simulink model "truesystem"  (R2020a)
settings: Solver=VariableStepAuto  StartTime=0.0  StopTime=stoptimetotal  RelTol=1e-3
values from neighbouring files (symbols this model uses):
  battery = load('params/battery.mat').battery    [prognostics.m]    (also in workspace_1.mat = )
  IC = load('params/IC_HoverAt10ftOcto.mat').IC    [prognostics.m]    (also in workspace_1.mat = )
  Motor1 = load('params/Motors/Motor1.mat').Motor    [prognostics.m]    (also in workspace_1.mat = )
  Motor2 = load('params/Motors/Motor2.mat').Motor    [prognostics.m]    (also in workspace_1.mat = )
  Motor3 = load('params/Motors/Motor3.mat').Motor    [prognostics.m]    (also in workspace_1.mat = )
  Motor4 = load('params/Motors/Motor4.mat').Motor    [prognostics.m]    (also in workspace_1.mat = )
  Motor5 = load('params/Motors/Motor5.mat').Motor    [prognostics.m]    (also in workspace_1.mat = )
  Motor6 = load('params/Motors/Motor6.mat').Motor    [prognostics.m]    (also in workspace_1.mat = )
  Motor7 = load('params/Motors/Motor7.mat').Motor    [prognostics.m]    (also in workspace_1.mat = )
  Motor8 = load('params/Motors/Motor8.mat').Motor    [prognostics.m]    (also in workspace_1.mat = )
  octomodel = load('params/octoModel.mat').octomodel    [prognostics.m]    (also in workspace_1.mat = )
  sampletimetraj = 1    [prognostics.m]    (also in workspace_1.mat)
undefined symbols (not defined in the file or in its folder): DiscIntNeverNeededParam, mu_wind
libraries: dspstat3 x9, sharedTrackingLibrary x4
(part 2 of 2)

== system truesystem/Motors/DC Motor 3/Mechanical part ==
  Static Friction Torque : Inport
  Electrical Torque : Inport  Port=2
  1/J Inertia constant : Gain  Gain=1/Motor3.J
  "Df viscous damping coefficient Dynamic Friction coefficient " : Gain  Gain=Motor3.Df
  Discrete-Time Integrator : DiscreteIntegrator  gainval=1  InitialCondition=IC.w3  SampleTime=octomodel.sampletime  ICPrevOutput=DiscIntNeverNeededParam  ICPrevScaledInput=DiscIntNeverNeededParam
  Gain : Gain  Gain=Motor3.cq
  Square : Math  Operator=square  SaturateOnIntegerOverflow=on
  Sum1 : Sum  Inputs=--+-
  w angular speed : Outport  VectorParamsAs1DForOutWhenUnconnected=off
  Torque : Outport  Port=2  VectorParamsAs1DForOutWhenUnconnected=off
  wires:
  1/J Inertia constant/1 -> Discrete-Time Integrator/1
  Static Friction Torque/1 -> Sum1/2
  "Df viscous damping coefficient Dynamic Friction coefficient "/1 -> Sum1/4
  Discrete-Time Integrator/1 -> w angular speed/1, Square/1, "Df viscous damping coefficient Dynamic Friction coefficient "/1  "w angular speed"
  Sum1/1 -> 1/J Inertia constant/1
  Electrical Torque/1 -> Sum1/3
  Gain/1 -> Torque/1, Sum1/1
  Square/1 -> Gain/1

== system truesystem/Motors/DC Motor 4/Electrical part ==
  ESC voltage : Inport
  w angular speed : Inport  Port=2
  1/R : Gain  Gain=1/Motor2.Req
  Ke (Torque constant)1 : Gain  Gain=Motor2.Ke_eq
  Kt (Torque constant) Kt=Ke for an ideal square wave motor : Gain  Gain=Motor2.Ke_eq
  Saturation : Saturate  UpperLimit=11  LowerLimit=0
  Scope1 : Scope
  Scope2 : Scope
  Scope3 : Scope
  Sum : Sum  Inputs=|+-
  Electrical Torque : Outport  VectorParamsAs1DForOutWhenUnconnected=off
  current : Outport  Port=2  VectorParamsAs1DForOutWhenUnconnected=off
  wires:
  Saturation/1 -> current/1, Kt (Torque constant) Kt=Ke for an ideal square wave motor/1, Scope1/1
  w angular speed/1 -> Ke (Torque constant)1/1
  ESC voltage/1 -> Sum/1
  Ke (Torque constant)1/1 -> Sum/2, Scope2/1
  Kt (Torque constant) Kt=Ke for an ideal square wave motor/1 -> Electrical Torque/1
  Sum/1 -> 1/R/1, Scope3/1
  1/R/1 -> Saturation/1  "current i"

== system truesystem/Motors/DC Motor 4/Mechanical part ==
  Static Friction Torque : Inport
  Electrical Torque : Inport  Port=2
  1/J Inertia constant : Gain  Gain=1/Motor2.J
  "Df viscous damping coefficient Dynamic Friction coefficient " : Gain  Gain=Motor2.Df
  Discrete-Time Integrator : DiscreteIntegrator  gainval=1  InitialCondition=IC.w2  SampleTime=octomodel.sampletime  ICPrevOutput=DiscIntNeverNeededParam  ICPrevScaledInput=DiscIntNeverNeededParam
  Gain : Gain  Gain=Motor2.cq
  Square : Math  Operator=square  SaturateOnIntegerOverflow=on
  Sum1 : Sum  Inputs=--+-
  w angular speed : Outport  VectorParamsAs1DForOutWhenUnconnected=off
  Torque : Outport  Port=2  VectorParamsAs1DForOutWhenUnconnected=off
  wires:
  Square/1 -> Gain/1
  Gain/1 -> Sum1/1, Torque/1
  Electrical Torque/1 -> Sum1/3
  Sum1/1 -> 1/J Inertia constant/1
  Discrete-Time Integrator/1 -> "Df viscous damping coefficient Dynamic Friction coefficient "/1, Square/1, w angular speed/1  "w angular speed"
  "Df viscous damping coefficient Dynamic Friction coefficient "/1 -> Sum1/4
  Static Friction Torque/1 -> Sum1/2
  1/J Inertia constant/1 -> Discrete-Time Integrator/1

== system truesystem/Motors/DC Motor 4/Simulink Function ==
  Input : Inport  PortDimensions=2
  Input1 : Inport  Port=2
  MotorMeasurementFcn4 : TriggerPort  TriggerType=function-call  IsSimulinkFunction=on  FunctionName=MotorMeasurementFcn4  VariantControl=(inherit)
  MATLAB Function : MATLAB Function  TreatAsAtomicUnit=on
  x : ArgIn  DisableCoverage=on  ArgumentName=x
  xNext : ArgOut  DisableCoverage=on  ArgumentName=xNext
  wires:
  x/1 -> MATLAB Function/1("x ")
  MATLAB Function/1(x) -> xNext/1
  Input/1 -> MATLAB Function/2(u)
  Input1/1 -> MATLAB Function/3(param)

== system truesystem/Motors/DC Motor 5/Electrical part ==
  ESC voltage : Inport
  w angular speed : Inport  Port=2
  1/R : Gain  Gain=1/Motor2.Req
  Ke (Torque constant)1 : Gain  Gain=Motor2.Ke_eq
  Kt (Torque constant) Kt=Ke for an ideal square wave motor : Gain  Gain=Motor2.Ke_eq
  Saturation : Saturate  UpperLimit=11  LowerLimit=0
  Scope1 : Scope
  Scope2 : Scope
  Scope3 : Scope
  Sum : Sum  Inputs=|+-
  Electrical Torque : Outport  VectorParamsAs1DForOutWhenUnconnected=off
  current : Outport  Port=2  VectorParamsAs1DForOutWhenUnconnected=off
  wires:
  Saturation/1 -> current/1, Kt (Torque constant) Kt=Ke for an ideal square wave motor/1, Scope1/1
  w angular speed/1 -> Ke (Torque constant)1/1
  ESC voltage/1 -> Sum/1
  Ke (Torque constant)1/1 -> Sum/2, Scope2/1
  Kt (Torque constant) Kt=Ke for an ideal square wave motor/1 -> Electrical Torque/1
  Sum/1 -> 1/R/1, Scope3/1
  1/R/1 -> Saturation/1  "current i"

== system truesystem/Motors/DC Motor 5/Mechanical part ==
  Static Friction Torque : Inport
  Electrical Torque : Inport  Port=2
  1/J Inertia constant : Gain  Gain=1/Motor2.J
  "Df viscous damping coefficient Dynamic Friction coefficient " : Gain  Gain=Motor2.Df
  Discrete-Time Integrator : DiscreteIntegrator  gainval=1  InitialCondition=IC.w2  SampleTime=octomodel.sampletime  ICPrevOutput=DiscIntNeverNeededParam  ICPrevScaledInput=DiscIntNeverNeededParam
  Gain : Gain  Gain=Motor2.cq
  Square : Math  Operator=square  SaturateOnIntegerOverflow=on
  Sum1 : Sum  Inputs=--+-
  w angular speed : Outport  VectorParamsAs1DForOutWhenUnconnected=off
  Torque : Outport  Port=2  VectorParamsAs1DForOutWhenUnconnected=off
  wires:
  Square/1 -> Gain/1
  Gain/1 -> Sum1/1, Torque/1
  Electrical Torque/1 -> Sum1/3
  Sum1/1 -> 1/J Inertia constant/1
  Discrete-Time Integrator/1 -> "Df viscous damping coefficient Dynamic Friction coefficient "/1, Square/1, w angular speed/1  "w angular speed"
  "Df viscous damping coefficient Dynamic Friction coefficient "/1 -> Sum1/4
  Static Friction Torque/1 -> Sum1/2
  1/J Inertia constant/1 -> Discrete-Time Integrator/1

== system truesystem/Motors/DC Motor 5/Simulink Function ==
  Input : Inport  PortDimensions=2
  Input1 : Inport  Port=2
  MotorMeasurementFcn5 : TriggerPort  TriggerType=function-call  IsSimulinkFunction=on  FunctionName=MotorMeasurementFcn5  VariantControl=(inherit)
  MATLAB Function : MATLAB Function  TreatAsAtomicUnit=on
  x : ArgIn  DisableCoverage=on  ArgumentName=x
  xNext : ArgOut  DisableCoverage=on  ArgumentName=xNext
  wires:
  x/1 -> MATLAB Function/1("x ")
  MATLAB Function/1(x) -> xNext/1
  Input/1 -> MATLAB Function/2(u)
  Input1/1 -> MATLAB Function/3(param)

== system truesystem/Motors/DC Motor 6/Electrical part ==
  ESC voltage : Inport
  w angular speed : Inport  Port=2
  1/R : Gain  Gain=1/Motor6.Req
  Ke (Torque constant)1 : Gain  Gain=Motor6.Ke_eq
  Kt (Torque constant) Kt=Ke for an ideal square wave motor : Gain  Gain=Motor6.Ke_eq
  Saturation : Saturate  UpperLimit=11  LowerLimit=0
  Sum : Sum  Inputs=|+-
  Electrical Torque : Outport  VectorParamsAs1DForOutWhenUnconnected=off
  current : Outport  Port=2  VectorParamsAs1DForOutWhenUnconnected=off
  wires:
  Saturation/1 -> current/1, Kt (Torque constant) Kt=Ke for an ideal square wave motor/1
  w angular speed/1 -> Ke (Torque constant)1/1
  ESC voltage/1 -> Sum/1
  Ke (Torque constant)1/1 -> Sum/2
  Kt (Torque constant) Kt=Ke for an ideal square wave motor/1 -> Electrical Torque/1
  Sum/1 -> 1/R/1
  1/R/1 -> Saturation/1  "current i"

== system truesystem/Motors/DC Motor 6/Mechanical part ==
  Static Friction Torque : Inport
  Electrical Torque : Inport  Port=2
  1/J Inertia constant : Gain  Gain=1/Motor6.J
  "Df viscous damping coefficient Dynamic Friction coefficient " : Gain  Gain=Motor6.Df
  Discrete-Time Integrator : DiscreteIntegrator  gainval=1  InitialCondition=IC.w6  SampleTime=octomodel.sampletime  ICPrevOutput=DiscIntNeverNeededParam  ICPrevScaledInput=DiscIntNeverNeededParam
  Gain : Gain  Gain=Motor6.cq
  Square : Math  Operator=square  SaturateOnIntegerOverflow=on
  Sum1 : Sum  Inputs=--+-
  w angular speed : Outport  VectorParamsAs1DForOutWhenUnconnected=off
  Torque : Outport  Port=2  VectorParamsAs1DForOutWhenUnconnected=off
  wires:
  Square/1 -> Gain/1
  Gain/1 -> Sum1/1, Torque/1
  Electrical Torque/1 -> Sum1/3
  Sum1/1 -> 1/J Inertia constant/1
  Discrete-Time Integrator/1 -> "Df viscous damping coefficient Dynamic Friction coefficient "/1, Square/1, w angular speed/1  "w angular speed"
  "Df viscous damping coefficient Dynamic Friction coefficient "/1 -> Sum1/4
  Static Friction Torque/1 -> Sum1/2
  1/J Inertia constant/1 -> Discrete-Time Integrator/1

== system truesystem/Motors/DC Motor 7/Electrical part ==
  ESC voltage : Inport
  w angular speed : Inport  Port=2
  1/R : Gain  Gain=1/Motor7.Req
  Ke (Torque constant)1 : Gain  Gain=Motor7.Ke_eq
  Kt (Torque constant) Kt=Ke for an ideal square wave motor : Gain  Gain=Motor7.Ke_eq
  Saturation : Saturate  UpperLimit=11  LowerLimit=0
  Sum : Sum  Inputs=|+-
  Electrical Torque : Outport  VectorParamsAs1DForOutWhenUnconnected=off
  current : Outport  Port=2  VectorParamsAs1DForOutWhenUnconnected=off
  wires:
  1/R/1 -> Saturation/1  "current i"
  Sum/1 -> 1/R/1
  Kt (Torque constant) Kt=Ke for an ideal square wave motor/1 -> Electrical Torque/1
  Ke (Torque constant)1/1 -> Sum/2
  ESC voltage/1 -> Sum/1
  w angular speed/1 -> Ke (Torque constant)1/1
  Saturation/1 -> Kt (Torque constant) Kt=Ke for an ideal square wave motor/1, current/1

== system truesystem/Motors/DC Motor 7/Mechanical part ==
  Static Friction Torque : Inport
  Electrical Torque : Inport  Port=2
  1/J Inertia constant : Gain  Gain=1/Motor7.J
  "Df viscous damping coefficient Dynamic Friction coefficient " : Gain  Gain=Motor7.Df
  Discrete-Time Integrator : DiscreteIntegrator  gainval=1  InitialCondition=IC.w7  SampleTime=octomodel.sampletime  ICPrevOutput=DiscIntNeverNeededParam  ICPrevScaledInput=DiscIntNeverNeededParam
  Gain : Gain  Gain=Motor7.cq
  Square : Math  Operator=square  SaturateOnIntegerOverflow=on
  Sum1 : Sum  Inputs=--+-
  w angular speed : Outport  VectorParamsAs1DForOutWhenUnconnected=off
  Torque : Outport  Port=2  VectorParamsAs1DForOutWhenUnconnected=off
  wires:
  1/J Inertia constant/1 -> Discrete-Time Integrator/1
  Static Friction Torque/1 -> Sum1/2
  "Df viscous damping coefficient Dynamic Friction coefficient "/1 -> Sum1/4
  Discrete-Time Integrator/1 -> w angular speed/1, Square/1, "Df viscous damping coefficient Dynamic Friction coefficient "/1  "w angular speed"
  Sum1/1 -> 1/J Inertia constant/1
  Electrical Torque/1 -> Sum1/3
  Gain/1 -> Torque/1, Sum1/1
  Square/1 -> Gain/1

== system truesystem/Motors/DC Motor 8/Electrical part ==
  ESC voltage : Inport
  w angular speed : Inport  Port=2
  1/R : Gain  Gain=1/Motor8.Req
  Ke (Torque constant)1 : Gain  Gain=Motor8.Ke_eq
  Kt (Torque constant) Kt=Ke for an ideal square wave motor : Gain  Gain=Motor8.Ke_eq
  Saturation : Saturate  UpperLimit=11  LowerLimit=0
  Sum : Sum  Inputs=|+-
  Electrical Torque : Outport  VectorParamsAs1DForOutWhenUnconnected=off
  current : Outport  Port=2  VectorParamsAs1DForOutWhenUnconnected=off
  wires:
  Saturation/1 -> current/1, Kt (Torque constant) Kt=Ke for an ideal square wave motor/1
  w angular speed/1 -> Ke (Torque constant)1/1
  ESC voltage/1 -> Sum/1
  Ke (Torque constant)1/1 -> Sum/2
  Kt (Torque constant) Kt=Ke for an ideal square wave motor/1 -> Electrical Torque/1
  Sum/1 -> 1/R/1
  1/R/1 -> Saturation/1  "current i"

== system truesystem/Motors/DC Motor 8/Mechanical part ==
  Static Friction Torque : Inport
  Electrical Torque : Inport  Port=2
  1/J Inertia constant : Gain  Gain=1/Motor8.J
  "Df viscous damping coefficient Dynamic Friction coefficient " : Gain  Gain=Motor8.Df
  Discrete-Time Integrator : DiscreteIntegrator  gainval=1  InitialCondition=IC.w8  SampleTime=octomodel.sampletime  ICPrevOutput=DiscIntNeverNeededParam  ICPrevScaledInput=DiscIntNeverNeededParam
  Gain : Gain  Gain=Motor8.cq
  Square : Math  Operator=square  SaturateOnIntegerOverflow=on
  Sum1 : Sum  Inputs=--+-
  w angular speed : Outport  VectorParamsAs1DForOutWhenUnconnected=off
  Torque : Outport  Port=2  VectorParamsAs1DForOutWhenUnconnected=off
  wires:
  Square/1 -> Gain/1
  Gain/1 -> Sum1/1, Torque/1
  Electrical Torque/1 -> Sum1/3
  Sum1/1 -> 1/J Inertia constant/1
  Discrete-Time Integrator/1 -> "Df viscous damping coefficient Dynamic Friction coefficient "/1, Square/1, w angular speed/1  "w angular speed"
  "Df viscous damping coefficient Dynamic Friction coefficient "/1 -> Sum1/4
  Static Friction Torque/1 -> Sum1/2
  1/J Inertia constant/1 -> Discrete-Time Integrator/1

== matlab function truesystem/Simulink Function/MATLAB Function ==
  data: x input; u input; x output
function x = positionTransitionFunction(x,u)

dt = 0.01; % [s] Sample time
x = x + fnContinuous(x,u)*dt;

end

function dxdt = fnContinuous(x,u)
g=9.8; % gravity acceleration
% States
x_pos= x(1);
y_pos= x(2); 
z_pos= x(3);  
V_x= x(4);
V_y= x(5);
V_z= x(6);
Phi= x(7);
The= x(8);
Psi= x(9);

% Inputs
a_x= u(1);
a_y= u(2);
a_z= u(3);
p= u(4);
q= u(5);
r= u(6);

R_b_e = [cos(Psi)*cos(The) cos(Psi)*sin(The)*sin(Phi)-sin(Psi)*cos(Phi) cos(Psi)*sin(The)*cos(Phi)+sin(Psi)*sin(Phi);
       sin(Psi)*cos(The) sin(Psi)*sin(The)*sin(Phi)+cos(Psi)*cos(Phi) sin(Psi)*sin(The)*cos(Phi)-cos(Psi)*sin(Phi);
       -sin(The)         cos(The)*sin(Phi)                            cos(The)*cos(Phi)]; % Rib

dxdt = [ V_x  ; ...
         V_y ; ...
         V_z ; ...
         cos(Psi)*cos(The)*a_x + (cos(Psi)*sin(The)*sin(Phi)-sin(Psi)*cos(Phi))*a_y + (cos(Psi)*sin(The)*cos(Phi)+sin(Psi)*sin(Phi))*a_z; ...
         sin(Psi)*cos(The)*a_x + (sin(Psi)*sin(The)*sin(Phi)+cos(Psi)*cos(Phi))*a_y + (sin(Psi)*sin(The)*cos(Phi)-cos(Psi)*sin(Phi))*a_z; ...
         -sin(The)*a_x + cos(The)*sin(Phi)*a_y + cos(The)*cos(Phi)*a_z ; ...%- g ; ...
         p + q*sin(Phi)*tan(The) + r*cos(Phi)*tan(The); ...
         q*cos(Phi) - r*sin(Phi) ; ...
         q*sin(Phi)/cos(The) + r*cos(Phi)/cos(The)];
end

== matlab function truesystem/Adding noise ==
  data: u input; y output; t input
function y = fcn(u,t)
if t==2.99
    see=1;
end
y = zeros(6,1);
% posnoisestd=0.75; % gives maximum and minimum of +-3 meters
posnoisestd=0.5; % gives maximum and minimum of +-2 meters
velnoisestd=0.025;
noisepos=posnoisestd.*randn(3,1);
noisevel=velnoisestd.*randn(3,1);
noise=[noisepos ;noisevel];
y = y + u + noise;

== matlab function truesystem/Motors/DC Motor 4/Simulink Function/MATLAB Function ==
  data: x input; u input; x output; param input
function x = MotorMeasurementFcn(x,u,param)

x = double(x*u(2) + param*u(1));

end

== matlab function truesystem/Motors/DC Motor 5/MATLAB Function ==
  settings: updateMethod=DISCRETE  sampleTime=.2
  data: mu input; y output; sigma input
function y = addNoise(mu, sigma)

y = normrnd(mu, sigma);

== matlab function truesystem/Motors/DC Motor 5/MATLAB Function1 ==
  settings: updateMethod=DISCRETE  sampleTime=.2
  data: mu input; y output; sigma input
function y = addNoise(mu, sigma)

y = normrnd(mu, sigma);

== matlab function truesystem/Motors/DC Motor 5/Simulink Function/MATLAB Function ==
  data: x input; u input; x output; param input
function x = MotorMeasurementFcn(x,u,param)

x = double(x*u(2) + param*u(1));

end

== matlab function truesystem/Subsystem/MATLAB Function2 ==
  settings: updateMethod=DISCRETE  sampleTime=.2
  data: mu input; y output; sigma input
function y = addNoise(mu, sigma)

y = normrnd(mu, sigma);

== matlab function truesystem/Subsystem/MATLAB Function1 ==
  settings: updateMethod=DISCRETE  sampleTime=.2
  data: mu input; y output; sigma input
function y = addNoise(mu, sigma)

y = normrnd(mu, sigma);

== matlab function truesystem/Motors/DC Motor 4/MATLAB Function ==
  settings: updateMethod=DISCRETE  sampleTime=.2
  data: mu input; y output; sigma input
function y = addNoise(mu, sigma)

y = normrnd(mu, sigma);

== matlab function truesystem/arrival condition ==
  data: currentpos input; arrived output; dest input
function arrived = fcn(currentpos,dest)

result=norm(currentpos-dest);
if result<1 % less than one meter from the goal
    arrived=1;
else
    arrived=0;
end

== matlab function truesystem/lowsoc ==
  data: soc input; lowsoc output; threshold input
function lowsoc = fcn(soc,threshold)


if soc<threshold % less than one meter from the goal
    lowsoc=1;
else
    lowsoc=0;
end

== matlab function truesystem/Motors/DC Motor 4/MATLAB Function1 ==
  settings: updateMethod=DISCRETE  sampleTime=.2
  data: mu input; y output; sigma input
function y = addNoise(mu, sigma)

y = normrnd(mu, sigma);

== matlab function truesystem/Motors/DC Motor 2/MATLAB Function ==
  settings: updateMethod=DISCRETE  sampleTime=.2
  data: mu input; y output; sigma input
function y = addNoise(mu, sigma)

y = normrnd(mu, sigma);

== matlab function truesystem/Motors/DC Motor 2/MATLAB Function1 ==
  settings: updateMethod=DISCRETE  sampleTime=.2
  data: mu input; y output; sigma input
function y = addNoise(mu, sigma)

y = normrnd(mu, sigma);

== matlab function truesystem/Control allocation ==
  data: Fx input; wref1 output; Fy input; Fz input; Troll input; Tpitch input; Tyaw input; wref2 output; wref3 output; wref4 output; wref5 output; wref6 output; wref7 output; wref8 output
function [wref1,wref2,wref3,wref4,wref5,wref6,wref7,wref8] = fcn(Fx,Fy,Fz,Troll,Tpitch,Tyaw)
%% parameters 
%Maximum speed that the motors can reach in rad/s, if I check voltage, I
%dont have to check speed
% Max_speed=710.31;
Max_speed=1000;

% arm length - distances from the octorotor center of mass ...
%        to the center of mass of all its rotors are equal and denoted by l.
l=0.35;
% thrust motor constant [Ns^2/rad^2]
b=8.54858e-06; % cq
% rotor drag constant [Nms^2/rad^2]
d=1.3678e-07; % ct
% control allocation matrix
A_f=[2*b 2*b 2*b 2*b; ...
    b*l 0 -b*l 0; ...
    -b*l -sqrt(2)*b*l b*l sqrt(2)*b*l; ...
    -2*d 2*d -2*d 2*d];
%desired input
u_des=[Fz;Troll;Tpitch;Tyaw];

%control allocation
Omega_sf=inv(A_f)*u_des;

%selection operator
E=[1 0 1 0 0 0 0 0;...
    0 1 0 1 0 0 0 0; ...
    0 0 0 0 1 0 1 0;...
    0 0 0 0 0 1 0 1]';

Omega_s=E*Omega_sf;

% velocity checking
wref=zeros(8);
for i=1:length(Omega_s)
    if Omega_s(i)<0
        wref(i)=0;
    elseif Omega_s(i)>Max_speed^2
        wref(i)=Max_speed;
    else
        wref(i)=sqrt(Omega_s(i));
    end
end

%velocity assignment in V
multiply=0.012240; %for 6783 rpm considering torque load 
for i=1:length(wref)
    % voltage saturation check
    if(wref(i)*multiply > 11.1)
        wref(i)=11.1;
    else
        wref(i)=wref(i)*multiply;
    end
end

wref1=wref(1);
wref2=wref(2);
wref3=wref(3);
wref4=wref(4);
wref5=wref(5);
wref6=wref(6);
wref7=wref(7);
wref8=wref(8);







% %% parameters required
% % load('params/octoModel.mat');
% gamma=3;%octomodel.tiltmotorangle;
% alpha=45;%octomodel.separationmotorangle;
% dl=0.45;%octomodel.dl;
% constant=(1/sqrt(2));
% ds=0.35;%octomodel.ds;
% ct=3.4262e-05;%octomodel.ct*(60/(2*pi))^2 -> in octomodel is for rpm, here I need it in rad/s;
% cq=9.3846e-07;%octomodel.cq*(60/(2*pi))^2 -> in octomodel is for rpm, here I need it in rad/s;
% 
% %% rotation matrices because of 3 degrees tilted angle
% 
% E_m_b = [0 -sin(alpha)*sin(gamma) sin(gamma) -cos(alpha)*sin(gamma) 0 sin(alpha)*sin(gamma) -sin(gamma) cos(alpha)*sin(gamma);
%          -sin(gamma)  cos(alpha)*sin(gamma) 0 -sin(alpha)*sin(gamma) sin(gamma) -cos(alpha)*sin(gamma) 0 sin(alpha)*sin(gamma);
%          -cos(gamma) -cos(gamma) -cos(gamma) -cos(gamma) -cos(gamma) -cos(gamma) -cos(gamma) -cos(gamma)];
% 
% R_m=[dl 0 0; ...
%     constant*ds constant*ds 0; ...
%     0 dl 0; ...
%     -constant*ds constant*ds 0; ...
%     -dl 0 0; ...
%     -constant*ds -constant*ds 0; ...
%     0 -dl 0; ...
%     constant*ds -constant*ds 0]';
% 
% %% first form delta_b matrix
% %a vectors
% a=zeros(3,8);
% for i=1:8
%     e_i_b=E_m_b(:,i);
%     a(:,i)=(ct).*e_i_b;
% end
% 
% %b vectors
% b=zeros(3,8);
% for i=1:8
%     e_i_b=E_m_b(:,i);
%     r_m=R_m(:,i);
%     b(:,i)=cross( r_m,(ct).*e_i_b ) + ((-1)^(i+1)*(cq)).*e_i_b;    
% end
% 
% %form matrix
% delta_b=[a;b];
% 
% %find pseudo-inverse
% delta_binv = pinv(delta_b);
% 
% %% calculate required w_ref
% Forces=[Fx,Fy,Fz];
% Torques=[Troll,Tpitch,Tyaw];
% if Troll>0
%     see=1;
% end
% input=[Forces,Torques]';
% wref=delta_binv*input;
% %check if complex
% if(isreal(wref(2)))
%     see=1;
% end
% 
% if length(find(wref<0))>0
%     pos=find(wref<0);
%     wref(pos)=0;
% end
% wref=sqrt(wref);
% 
% % %angular velocity in rad/s
% % wref1=wref(1);
% % wref2=wref(2);
% % wref3=wref(3);
% % wref4=wref(4);
% % wref5=wref(5);
% % wref6=wref(6);
% % wref7=wref(7);
% % wref8=wref(8);
% 
% %angular velocity in rpm
% % wref1=wref(1)*(60/(2*pi));
% % wref2=wref(2)*(60/(2*pi));
% % wref3=wref(3)*(60/(2*pi));
% % wref4=wref(4)*(60/(2*pi));
% % wref5=wref(5)*(60/(2*pi));
% % wref6=wref(6)*(60/(2*pi));
% % wref7=wref(7)*(60/(2*pi));
% % wref8=wref(8)*(60/(2*pi));
% 
% %% now convert to voltage in the range 0-22V
% % divide=36.17; %true is 36.37
% % multiply=0.0238; %for 8800 rpm nominal 
% multiply=0.02762; %for 6783 rpm considering torque load 
% wref1=wref(1)*multiply;
% wref2=wref(2)*multiply;
% wref3=wref(3)*multiply;
% wref4=wref(4)*multiply;
% wref5=wref(5)*multiply;
% wref6=wref(6)*multiply;
% wref7=wref(7)*multiply;
% wref8=wref(8)*multiply;
% 
% see=1;

end

== matlab function truesystem/Motors/DC Motor 2/Simulink Function/MATLAB Function ==
  data: x input; u input; x output; param input
function x = MotorMeasurementFcn(x,u,param)

x = double(x*u(2) + param*u(1));

end
